simulink model "x5_Click"  (R2024b)
settings: Solver=VariableStepAuto  StartTime=0.0  StopTime=inf  RelTol=1e-3  EnableMultiTasking=on
libraries: simulink x6
(part 1 of 3)
settings Model: Creator=jorgemartins  LastModifiedBy=pinto
settings SolverCC: AlgebraicLoopSolver=TrustRegion
settings DataIOCC: LimitDataPoints=on  ReturnWorkspaceOutputs=off
settings OptimizationCC: LifeSpan=inf
settings DebuggingCC: UnconnectedInputMsg=warning  UnconnectedOutputMsg=warning  UnconnectedLineMsg=warning  AllowSymbolicDim=off  SFUnexpectedBacktrackingDiag=warning  SFNoUnconditionalDefaultTransitionDiag=warning  SFExecutionAtInitializationDiag=none  ArithmeticOperatorsInVariantConditions=warning
settings ModelReferenceCC: EnableRefExpFcnMdlSchedulingChecks=on  PropagateSignalLabelsOutOfModel=off
settings SFSimCC: SimUseLocalCustomCode=off  CustomCodeUndefinedFunction=UseInterfaceOnly
settings RTWCC: RTWUseLocalCustomCode=off  GPUComputeCapability=3.5
settings CodeAppCC: StateflowObjectComments=on
settings GRTTargetCC: TargetLangStandard=C89/C90 (ANSI)
settings ConfigComp: CovMetricSettings=dw  CovSaveCumulativeToWorkspaceVar=on  CovSaveSingleToWorkspaceVar=on  CovExternalEMLEnable=off

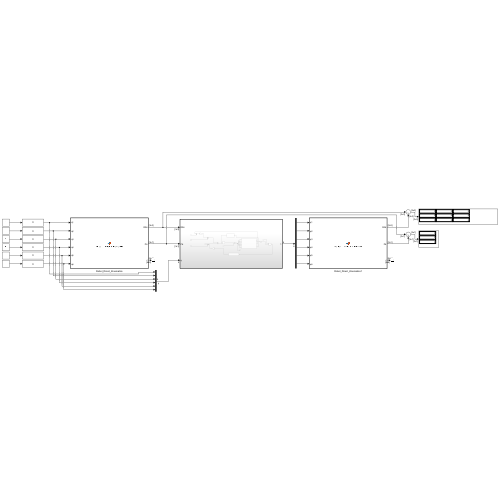
[thumbnail: Simulink's stored preview of the top-level diagram]
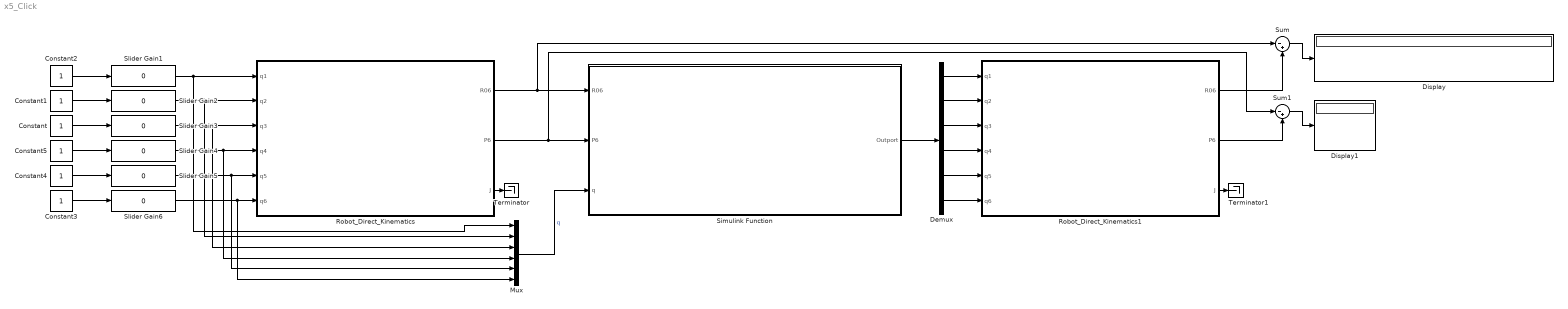
== system x5_Click ==
  Constant{,1..5} (6 alike) : Constant
  Demux : Demux  Outputs=6
  Display : Display
  Display1 : Display
  Mux : Mux  Inputs=6
  Robot_Direct_Kinematics : MATLAB Function  TreatAsAtomicUnit=on
  Robot_Direct_Kinematics1 : MATLAB Function  TreatAsAtomicUnit=on
  Simulink Function : Subsystem  TreatAsAtomicUnit=on
  Slider Gain1 : simulink/Math Operations/Slider Gain  gain=0  low=-3.14  high=0
  Slider Gain{2..4,6} (4 alike) : simulink/Math Operations/Slider Gain  gain=0  low=-3.14  high=3.14
  Slider Gain5 : simulink/Math Operations/Slider Gain  gain=0  low=-3.14  high=0
  Sum : Sum  Inputs=|-+
  Sum1 : Sum  Inputs=|-+
  Terminator : Terminator
  Terminator1 : Terminator
  wires:
  Slider Gain2/1 -> Mux/2, Robot_Direct_Kinematics/2(q2)
  Slider Gain3/1 -> Robot_Direct_Kinematics/3(q3), Mux/3
  Mux/1 -> Simulink Function/3(q)  "q"
  Slider Gain4/1 -> Mux/4, Robot_Direct_Kinematics/4(q4)
  Slider Gain1/1 -> Robot_Direct_Kinematics/1(q1), Mux/1
  Slider Gain5/1 -> Mux/5, Robot_Direct_Kinematics/5(q5)
  Slider Gain6/1 -> Mux/6, Robot_Direct_Kinematics/6(q6)
  Robot_Direct_Kinematics/1(R06) -> Sum/1, Simulink Function/1(R06)
  Robot_Direct_Kinematics/2(P6) -> Sum1/1, Simulink Function/2(P6)
  Constant/1 -> Slider Gain3/1
  Constant1/1 -> Slider Gain2/1
  Constant4/1 -> Slider Gain5/1
  Constant5/1 -> Slider Gain4/1
  Constant3/1 -> Slider Gain6/1
  Constant2/1 -> Slider Gain1/1
  Simulink Function/1(Outport) -> Demux/1
  Demux/1 -> Robot_Direct_Kinematics1/1(q1)
  Demux/2 -> Robot_Direct_Kinematics1/2(q2)
  Demux/3 -> Robot_Direct_Kinematics1/3(q3)
  Demux/4 -> Robot_Direct_Kinematics1/4(q4)
  Demux/5 -> Robot_Direct_Kinematics1/5(q5)
  Demux/6 -> Robot_Direct_Kinematics1/6(q6)
  Robot_Direct_Kinematics1/1(R06) -> Sum/2
  Robot_Direct_Kinematics1/2(P6) -> Sum1/2
  Sum/1 -> Display/1
  Sum1/1 -> Display1/1
  Robot_Direct_Kinematics/3(J) -> Terminator/1
  Robot_Direct_Kinematics1/3(J) -> Terminator1/1

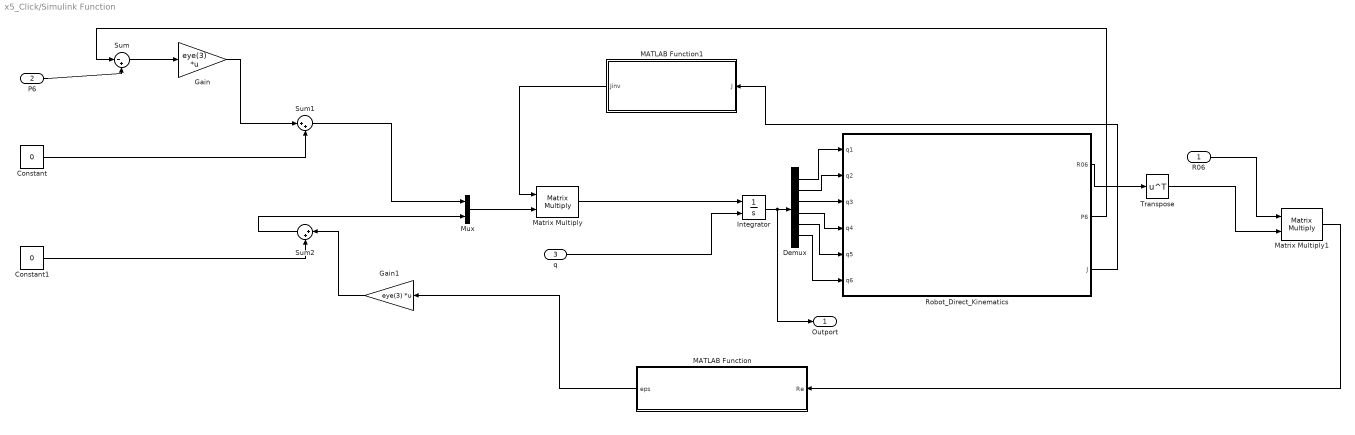
== system x5_Click/Simulink Function ==
  R06 : Inport
  P6 : Inport  Port=2
  q : Inport  Port=3
  Constant : Constant  Value=0
  Constant1 : Constant  Value=0
  Demux : Demux  Outputs=6
  Gain : Gain  Gain=eye(3)  Multiplication=Matrix(K*u) (u vector)
  Gain1 : Gain  Gain=eye(3)  Multiplication=Matrix(K*u) (u vector)
  Integrator : Integrator  InitialConditionSource=external
  MATLAB Function : MATLAB Function  TreatAsAtomicUnit=on
  MATLAB Function1 : MATLAB Function  TreatAsAtomicUnit=on
  Matrix Multiply : Product  Multiplication=Matrix(*)
  Matrix Multiply1 : Product  Multiplication=Matrix(*)
  Mux : Mux  Inputs=2
  Robot_Direct_Kinematics : MATLAB Function  TreatAsAtomicUnit=on
  Sum : Sum  Inputs=|-+
  Sum1 : Sum  Inputs=|++
  Sum2 : Sum  Inputs=|++
  Transpose : Math  Operator=transpose
  Outport : Outport
  wires:
  P6/1 -> Sum/2
  Sum/1 -> Gain/1
  Constant/1 -> Sum1/2
  Gain/1 -> Sum1/1
  Constant1/1 -> Sum2/2
  Gain1/1 -> Sum2/1
  Sum2/1 -> Mux/2
  Sum1/1 -> Mux/1
  Mux/1 -> Matrix Multiply/2
  q/1 -> Integrator/2
  Matrix Multiply/1 -> Integrator/1
  Integrator/1 -> Outport/1, Demux/1
  Demux/1 -> Robot_Direct_Kinematics/1(q1)
  Demux/2 -> Robot_Direct_Kinematics/2(q2)
  Demux/3 -> Robot_Direct_Kinematics/3(q3)
  Demux/4 -> Robot_Direct_Kinematics/4(q4)
  Demux/5 -> Robot_Direct_Kinematics/5(q5)
  Demux/6 -> Robot_Direct_Kinematics/6(q6)
  Robot_Direct_Kinematics/3(J) -> MATLAB Function1/1(J)
  Robot_Direct_Kinematics/2(P6) -> Sum/1
  R06/1 -> Matrix Multiply1/1
  Robot_Direct_Kinematics/1(R06) -> Transpose/1
  Transpose/1 -> Matrix Multiply1/2
  Matrix Multiply1/1 -> MATLAB Function/1(Re)
  MATLAB Function/1(eps) -> Gain1/1
  MATLAB Function1/1(Jinv) -> Matrix Multiply/1

== matlab function x5_Click/Simulink Function/Robot_Direct_Kinematics ==
  data: q1 input; R06 output; q2 input; q3 input; q4 input; q5 input; q6 input; P6 output; J output
function [R06,P6,J] = Robot_Direct_Kinematics(q1,q2,q3,q4,q5,q6)
%#codegen

%    This function was generated by the Symbolic Math Toolbox version 24.2.
%    21-May-2025 19:19:44

% q1 = complex(q1);  % if required to enforce complex operations
% q2 = complex(q2);  % if required to enforce complex operations
% q3 = complex(q3);  % if required to enforce complex operations
% q4 = complex(q4);  % if required to enforce complex operations
% q5 = complex(q5);  % if required to enforce complex operations
% q6 = complex(q6);  % if required to enforce complex operations
et1 = cos(q5).*sin(q1).*sin(q3).*sqrt(sqrt(2.0)+2.0).*(-1.0./2.0)-(cos(q1).*cos(q2).*sin(q4).*sin(q6).*sqrt(-sqrt(2.0)+2.0))./2.0-(cos(q3).*cos(q4).*sin(q1).*sin(q6).*sqrt(-sqrt(2.0)+2.0))./2.0-(cos(q6).*sin(q1).*sin(q3).*sin(q5).*sqrt(-sqrt(2.0)+2.0))./2.0-(cos(q1).*cos(q3).*cos(q5).*sin(q2).*sqrt(sqrt(2.0)+2.0))./2.0-(cos(q1).*cos(q2).*cos(q4).*sin(q5).*sqrt(sqrt(2.0)+2.0))./2.0+(cos(q3).*sin(q1).*sin(q4).*sin(q5).*sqrt(sqrt(2.0)+2.0))./2.0;
et2 = (cos(q1).*cos(q2).*cos(q4).*cos(q5).*cos(q6).*sqrt(-sqrt(2.0)+2.0))./2.0-(cos(q1).*cos(q3).*cos(q6).*sin(q2).*sin(q5).*sqrt(-sqrt(2.0)+2.0))./2.0-(cos(q3).*cos(q5).*cos(q6).*sin(q1).*sin(q4).*sqrt(-sqrt(2.0)+2.0))./2.0+(cos(q1).*cos(q4).*sin(q2).*sin(q3).*sin(q6).*sqrt(-sqrt(2.0)+2.0))./2.0-(cos(q1).*sin(q2).*sin(q3).*sin(q4).*sin(q5).*sqrt(sqrt(2.0)+2.0))./2.0+(cos(q1).*cos(q5).*cos(q6).*sin(q2).*sin(q3).*sin(q4).*sqrt(-sqrt(2.0)+2.0))./2.0;
et3 = cos(q1).*cos(q5).*sin(q3).*sqrt(sqrt(2.0)+2.0).*(-1.0./2.0)-(cos(q1).*cos(q3).*cos(q4).*sin(q6).*sqrt(-sqrt(2.0)+2.0))./2.0-(cos(q1).*cos(q6).*sin(q3).*sin(q5).*sqrt(-sqrt(2.0)+2.0))./2.0+(cos(q2).*sin(q1).*sin(q4).*sin(q6).*sqrt(-sqrt(2.0)+2.0))./2.0+(cos(q3).*cos(q5).*sin(q1).*sin(q2).*sqrt(sqrt(2.0)+2.0))./2.0+(cos(q2).*cos(q4).*sin(q1).*sin(q5).*sqrt(sqrt(2.0)+2.0))./2.0+(cos(q1).*cos(q3).*sin(q4).*sin(q5).*sqrt(sqrt(2.0)+2.0))./2.0-(cos(q2).*cos(q4).*cos(q5).*cos(q6).*sin(q1).*sqrt(-sqrt(2.0)+2.0))./2.0;
et4 = cos(q1).*cos(q3).*cos(q5).*cos(q6).*sin(q4).*sqrt(-sqrt(2.0)+2.0).*(-1.0./2.0)+(cos(q3).*cos(q6).*sin(q1).*sin(q2).*sin(q5).*sqrt(-sqrt(2.0)+2.0))./2.0-(cos(q4).*sin(q1).*sin(q2).*sin(q3).*sin(q6).*sqrt(-sqrt(2.0)+2.0))./2.0+(sin(q1).*sin(q2).*sin(q3).*sin(q4).*sin(q5).*sqrt(sqrt(2.0)+2.0))./2.0-(cos(q5).*cos(q6).*sin(q1).*sin(q2).*sin(q3).*sin(q4).*sqrt(-sqrt(2.0)+2.0))./2.0;
et5 = cos(q5).*sin(q1).*sin(q3).*sqrt(-sqrt(2.0)+2.0).*(-1.0./2.0)-(cos(q1).*cos(q3).*cos(q5).*sin(q2).*sqrt(-sqrt(2.0)+2.0))./2.0-(cos(q1).*cos(q2).*cos(q4).*sin(q5).*sqrt(-sqrt(2.0)+2.0))./2.0+(cos(q3).*sin(q1).*sin(q4).*sin(q5).*sqrt(-sqrt(2.0)+2.0))./2.0+(cos(q1).*cos(q2).*sin(q4).*sin(q6).*sqrt(sqrt(2.0)+2.0))./2.0+(cos(q3).*cos(q4).*sin(q1).*sin(q6).*sqrt(sqrt(2.0)+2.0))./2.0+(cos(q6).*sin(q1).*sin(q3).*sin(q5).*sqrt(sqrt(2.0)+2.0))./2.0;
et6 = cos(q1).*sin(q2).*sin(q3).*sin(q4).*sin(q5).*sqrt(-sqrt(2.0)+2.0).*(-1.0./2.0)-(cos(q1).*cos(q2).*cos(q4).*cos(q5).*cos(q6).*sqrt(sqrt(2.0)+2.0))./2.0+(cos(q1).*cos(q3).*cos(q6).*sin(q2).*sin(q5).*sqrt(sqrt(2.0)+2.0))./2.0+(cos(q3).*cos(q5).*cos(q6).*sin(q1).*sin(q4).*sqrt(sqrt(2.0)+2.0))./2.0-(cos(q1).*cos(q4).*sin(q2).*sin(q3).*sin(q6).*sqrt(sqrt(2.0)+2.0))./2.0-(cos(q1).*cos(q5).*cos(q6).*sin(q2).*sin(q3).*sin(q4).*sqrt(sqrt(2.0)+2.0))./2.0;
et7 = cos(q1).*cos(q5).*sin(q3).*sqrt(-sqrt(2.0)+2.0).*(-1.0./2.0)+(cos(q3).*cos(q5).*sin(q1).*sin(q2).*sqrt(-sqrt(2.0)+2.0))./2.0+(cos(q2).*cos(q4).*sin(q1).*sin(q5).*sqrt(-sqrt(2.0)+2.0))./2.0+(cos(q1).*cos(q3).*sin(q4).*sin(q5).*sqrt(-sqrt(2.0)+2.0))./2.0+(cos(q1).*cos(q3).*cos(q4).*sin(q6).*sqrt(sqrt(2.0)+2.0))./2.0+(cos(q1).*cos(q6).*sin(q3).*sin(q5).*sqrt(sqrt(2.0)+2.0))./2.0-(cos(q2).*sin(q1).*sin(q4).*sin(q6).*sqrt(sqrt(2.0)+2.0))./2.0;
et8 = (sin(q1).*sin(q2).*sin(q3).*sin(q4).*sin(q5).*sqrt(-sqrt(2.0)+2.0))./2.0+(cos(q2).*cos(q4).*cos(q5).*cos(q6).*sin(q1).*sqrt(sqrt(2.0)+2.0))./2.0+(cos(q1).*cos(q3).*cos(q5).*cos(q6).*sin(q4).*sqrt(sqrt(2.0)+2.0))./2.0-(cos(q3).*cos(q6).*sin(q1).*sin(q2).*sin(q5).*sqrt(sqrt(2.0)+2.0))./2.0+(cos(q4).*sin(q1).*sin(q2).*sin(q3).*sin(q6).*sqrt(sqrt(2.0)+2.0))./2.0+(cos(q5).*cos(q6).*sin(q1).*sin(q2).*sin(q3).*sin(q4).*sqrt(sqrt(2.0)+2.0))./2.0;
mt1 = [cos(q1).*cos(q3).*cos(q4).*cos(q6)-cos(q2).*cos(q6).*sin(q1).*sin(q4)-cos(q1).*sin(q3).*sin(q5).*sin(q6)-cos(q2).*cos(q4).*cos(q5).*sin(q1).*sin(q6)-cos(q1).*cos(q3).*cos(q5).*sin(q4).*sin(q6)+cos(q4).*cos(q6).*sin(q1).*sin(q2).*sin(q3)+cos(q3).*sin(q1).*sin(q2).*sin(q5).*sin(q6)-cos(q5).*sin(q1).*sin(q2).*sin(q3).*sin(q4).*sin(q6),cos(q1).*cos(q2).*cos(q6).*sin(q4)+cos(q3).*cos(q4).*cos(q6).*sin(q1)-sin(q1).*sin(q3).*sin(q5).*sin(q6)+cos(q1).*cos(q2).*cos(q4).*cos(q5).*sin(q6)-cos(q1).*cos(q4).*cos(q6).*sin(q2).*sin(q3)-cos(q1).*cos(q3).*sin(q2).*sin(q5).*sin(q6)-cos(q3).*cos(q5).*sin(q1).*sin(q4).*sin(q6)+cos(q1).*cos(q5).*sin(q2).*sin(q3).*sin(q4).*sin(q6)];
mt2 = [cos(q6).*sin(q2).*sin(q4)+cos(q2).*cos(q4).*cos(q6).*sin(q3)+cos(q2).*cos(q3).*sin(q5).*sin(q6)+cos(q4).*cos(q5).*sin(q2).*sin(q6)-cos(q2).*cos(q5).*sin(q3).*sin(q4).*sin(q6),et3+et4,et1+et2];
mt3 = [cos(q4).*sin(q2).*sin(q5).*sqrt(sqrt(2.0)+2.0).*(-1.0./2.0)-(sin(q2).*sin(q4).*sin(q6).*sqrt(-sqrt(2.0)+2.0))./2.0+(cos(q2).*cos(q3).*cos(q5).*sqrt(sqrt(2.0)+2.0))./2.0+(cos(q2).*cos(q3).*cos(q6).*sin(q5).*sqrt(-sqrt(2.0)+2.0))./2.0+(cos(q4).*cos(q5).*cos(q6).*sin(q2).*sqrt(-sqrt(2.0)+2.0))./2.0-(cos(q2).*cos(q4).*sin(q3).*sin(q6).*sqrt(-sqrt(2.0)+2.0))./2.0+(cos(q2).*sin(q3).*sin(q4).*sin(q5).*sqrt(sqrt(2.0)+2.0))./2.0-(cos(q2).*cos(q5).*cos(q6).*sin(q3).*sin(q4).*sqrt(-sqrt(2.0)+2.0))./2.0];
mt4 = [et7+et8,et5+et6,(sin(q2).*sin(q4).*sin(q6).*sqrt(sqrt(2.0)+2.0))./2.0+(cos(q2).*cos(q3).*cos(q5).*sqrt(-sqrt(2.0)+2.0))./2.0-(cos(q4).*sin(q2).*sin(q5).*sqrt(-sqrt(2.0)+2.0))./2.0+(cos(q2).*sin(q3).*sin(q4).*sin(q5).*sqrt(-sqrt(2.0)+2.0))./2.0-(cos(q2).*cos(q3).*cos(q6).*sin(q5).*sqrt(sqrt(2.0)+2.0))./2.0-(cos(q4).*cos(q5).*cos(q6).*sin(q2).*sqrt(sqrt(2.0)+2.0))./2.0+(cos(q2).*cos(q4).*sin(q3).*sin(q6).*sqrt(sqrt(2.0)+2.0))./2.0+(cos(q2).*cos(q5).*cos(q6).*sin(q3).*sin(q4).*sqrt(sqrt(2.0)+2.0))./2.0];
R06 = reshape([mt1,mt2,mt3,mt4],3,3);
if nargout > 1
    et9 = sin(q2).*(-2.0./5.0)+(cos(q4).*sin(q2))./1.0e+1+(sin(q2).*sin(q4))./2.0+(cos(q2).*cos(q3).*cos(q5))./1.0e+1+(cos(q2).*cos(q4).*sin(q3))./2.0-(cos(q2).*sin(q3).*sin(q4))./1.0e+1-(cos(q4).*sin(q2).*sin(q5))./1.0e+1+sin(q2).*sin(q4).*sin(q6).*sqrt(sqrt(2.0)+2.0).*(3.0./4.0e+1)+cos(q2).*cos(q3).*cos(q5).*sqrt(-sqrt(2.0)+2.0).*(3.0./4.0e+1)-cos(q4).*sin(q2).*sin(q5).*sqrt(-sqrt(2.0)+2.0).*(3.0./4.0e+1)+(cos(q2).*sin(q3).*sin(q4).*sin(q5))./1.0e+1+cos(q2).*sin(q3).*sin(q4).*sin(q5).*sqrt(-sqrt(2.0)+2.0).*(3.0./4.0e+1);
    et10 = cos(q2).*cos(q3).*cos(q6).*sin(q5).*sqrt(sqrt(2.0)+2.0).*(-3.0./4.0e+1)-cos(q4).*cos(q5).*cos(q6).*sin(q2).*sqrt(sqrt(2.0)+2.0).*(3.0./4.0e+1)+cos(q2).*cos(q4).*sin(q3).*sin(q6).*sqrt(sqrt(2.0)+2.0).*(3.0./4.0e+1)+cos(q2).*cos(q5).*cos(q6).*sin(q3).*sin(q4).*sqrt(sqrt(2.0)+2.0).*(3.0./4.0e+1);
    et11 = cos(q1).*cos(q2).*(-2.0./5.0)+(cos(q1).*cos(q2).*cos(q4))./1.0e+1+(cos(q1).*cos(q2).*sin(q4))./2.0+(cos(q3).*cos(q4).*sin(q1))./2.0-(cos(q3).*sin(q1).*sin(q4))./1.0e+1-(cos(q5).*sin(q1).*sin(q3))./1.0e+1-cos(q5).*sin(q1).*sin(q3).*sqrt(-sqrt(2.0)+2.0).*(3.0./4.0e+1)-(cos(q1).*cos(q3).*cos(q5).*sin(q2))./1.0e+1-(cos(q1).*cos(q2).*cos(q4).*sin(q5))./1.0e+1-(cos(q1).*cos(q4).*sin(q2).*sin(q3))./2.0+(cos(q1).*sin(q2).*sin(q3).*sin(q4))./1.0e+1+(cos(q3).*sin(q1).*sin(q4).*sin(q5))./1.0e+1-cos(q1).*cos(q3).*cos(q5).*sin(q2).*sqrt(-sqrt(2.0)+2.0).*(3.0./4.0e+1);
    et12 = cos(q1).*cos(q2).*cos(q4).*sin(q5).*sqrt(-sqrt(2.0)+2.0).*(-3.0./4.0e+1)+cos(q3).*sin(q1).*sin(q4).*sin(q5).*sqrt(-sqrt(2.0)+2.0).*(3.0./4.0e+1)-(cos(q1).*sin(q2).*sin(q3).*sin(q4).*sin(q5))./1.0e+1+cos(q1).*cos(q2).*sin(q4).*sin(q6).*sqrt(sqrt(2.0)+2.0).*(3.0./4.0e+1)+cos(q3).*cos(q4).*sin(q1).*sin(q6).*sqrt(sqrt(2.0)+2.0).*(3.0./4.0e+1)+cos(q6).*sin(q1).*sin(q3).*sin(q5).*sqrt(sqrt(2.0)+2.0).*(3.0./4.0e+1)-cos(q1).*sin(q2).*sin(q3).*sin(q4).*sin(q5).*sqrt(-sqrt(2.0)+2.0).*(3.0./4.0e+1)-cos(q1).*cos(q2).*cos(q4).*cos(q5).*cos(q6).*sqrt(sqrt(2.0)+2.0).*(3.0./4.0e+1);
    et13 = cos(q1).*cos(q3).*cos(q6).*sin(q2).*sin(q5).*sqrt(sqrt(2.0)+2.0).*(3.0./4.0e+1)+cos(q3).*cos(q5).*cos(q6).*sin(q1).*sin(q4).*sqrt(sqrt(2.0)+2.0).*(3.0./4.0e+1)-cos(q1).*cos(q4).*sin(q2).*sin(q3).*sin(q6).*sqrt(sqrt(2.0)+2.0).*(3.0./4.0e+1)-cos(q1).*cos(q5).*cos(q6).*sin(q2).*sin(q3).*sin(q4).*sqrt(sqrt(2.0)+2.0).*(3.0./4.0e+1);
    et14 = cos(q2).*sin(q1).*(2.0./5.0)+(cos(q1).*cos(q3).*cos(q4))./2.0-(cos(q2).*cos(q4).*sin(q1))./1.0e+1-(cos(q1).*cos(q3).*sin(q4))./1.0e+1-(cos(q1).*cos(q5).*sin(q3))./1.0e+1-(cos(q2).*sin(q1).*sin(q4))./2.0-cos(q1).*cos(q5).*sin(q3).*sqrt(-sqrt(2.0)+2.0).*(3.0./4.0e+1)+(cos(q3).*cos(q5).*sin(q1).*sin(q2))./1.0e+1+(cos(q2).*cos(q4).*sin(q1).*sin(q5))./1.0e+1+(cos(q1).*cos(q3).*sin(q4).*sin(q5))./1.0e+1+(cos(q4).*sin(q1).*sin(q2).*sin(q3))./2.0-(sin(q1).*sin(q2).*sin(q3).*sin(q4))./1.0e+1+cos(q3).*cos(q5).*sin(q1).*sin(q2).*sqrt(-sqrt(2.0)+2.0).*(3.0./4.0e+1);
    et15 = cos(q2).*cos(q4).*sin(q1).*sin(q5).*sqrt(-sqrt(2.0)+2.0).*(3.0./4.0e+1)+cos(q1).*cos(q3).*sin(q4).*sin(q5).*sqrt(-sqrt(2.0)+2.0).*(3.0./4.0e+1)+(sin(q1).*sin(q2).*sin(q3).*sin(q4).*sin(q5))./1.0e+1+cos(q1).*cos(q3).*cos(q4).*sin(q6).*sqrt(sqrt(2.0)+2.0).*(3.0./4.0e+1)+cos(q1).*cos(q6).*sin(q3).*sin(q5).*sqrt(sqrt(2.0)+2.0).*(3.0./4.0e+1)-cos(q2).*sin(q1).*sin(q4).*sin(q6).*sqrt(sqrt(2.0)+2.0).*(3.0./4.0e+1)+sin(q1).*sin(q2).*sin(q3).*sin(q4).*sin(q5).*sqrt(-sqrt(2.0)+2.0).*(3.0./4.0e+1)+cos(q2).*cos(q4).*cos(q5).*cos(q6).*sin(q1).*sqrt(sqrt(2.0)+2.0).*(3.0./4.0e+1);
    et16 = cos(q1).*cos(q3).*cos(q5).*cos(q6).*sin(q4).*sqrt(sqrt(2.0)+2.0).*(3.0./4.0e+1)-cos(q3).*cos(q6).*sin(q1).*sin(q2).*sin(q5).*sqrt(sqrt(2.0)+2.0).*(3.0./4.0e+1)+cos(q4).*sin(q1).*sin(q2).*sin(q3).*sin(q6).*sqrt(sqrt(2.0)+2.0).*(3.0./4.0e+1)+cos(q5).*cos(q6).*sin(q1).*sin(q2).*sin(q3).*sin(q4).*sqrt(sqrt(2.0)+2.0).*(3.0./4.0e+1);
    P6 = [et14+et15+et16;et11+et12+et13;et9+et10];
end
if nargout > 2
    et17 = cos(q2).*sin(q1).*(2.0./5.0)+(cos(q1).*cos(q3).*cos(q4))./2.0-(cos(q2).*cos(q4).*sin(q1))./1.0e+1-(cos(q1).*cos(q3).*sin(q4))./1.0e+1-(cos(q1).*cos(q5).*sin(q3))./1.0e+1-(cos(q2).*sin(q1).*sin(q4))./2.0-cos(q1).*cos(q5).*sin(q3).*sqrt(-sqrt(2.0)+2.0).*(3.0./4.0e+1)+(cos(q3).*cos(q5).*sin(q1).*sin(q2))./1.0e+1+(cos(q2).*cos(q4).*sin(q1).*sin(q5))./1.0e+1+(cos(q1).*cos(q3).*sin(q4).*sin(q5))./1.0e+1+(cos(q4).*sin(q1).*sin(q2).*sin(q3))./2.0-(sin(q1).*sin(q2).*sin(q3).*sin(q4))./1.0e+1+cos(q3).*cos(q5).*sin(q1).*sin(q2).*sqrt(-sqrt(2.0)+2.0).*(3.0./4.0e+1);
    et18 = cos(q2).*cos(q4).*sin(q1).*sin(q5).*sqrt(-sqrt(2.0)+2.0).*(3.0./4.0e+1)+cos(q1).*cos(q3).*sin(q4).*sin(q5).*sqrt(-sqrt(2.0)+2.0).*(3.0./4.0e+1)+(sin(q1).*sin(q2).*sin(q3).*sin(q4).*sin(q5))./1.0e+1+cos(q1).*cos(q3).*cos(q4).*sin(q6).*sqrt(sqrt(2.0)+2.0).*(3.0./4.0e+1)+cos(q1).*cos(q6).*sin(q3).*sin(q5).*sqrt(sqrt(2.0)+2.0).*(3.0./4.0e+1)-cos(q2).*sin(q1).*sin(q4).*sin(q6).*sqrt(sqrt(2.0)+2.0).*(3.0./4.0e+1)+sin(q1).*sin(q2).*sin(q3).*sin(q4).*sin(q5).*sqrt(-sqrt(2.0)+2.0).*(3.0./4.0e+1)+cos(q2).*cos(q4).*cos(q5).*cos(q6).*sin(q1).*sqrt(sqrt(2.0)+2.0).*(3.0./4.0e+1);
    et19 = cos(q1).*cos(q3).*cos(q5).*cos(q6).*sin(q4).*sqrt(sqrt(2.0)+2.0).*(3.0./4.0e+1)-cos(q3).*cos(q6).*sin(q1).*sin(q2).*sin(q5).*sqrt(sqrt(2.0)+2.0).*(3.0./4.0e+1)+cos(q4).*sin(q1).*sin(q2).*sin(q3).*sin(q6).*sqrt(sqrt(2.0)+2.0).*(3.0./4.0e+1)+cos(q5).*cos(q6).*sin(q1).*sin(q2).*sin(q3).*sin(q4).*sqrt(sqrt(2.0)+2.0).*(3.0./4.0e+1);
    et20 = cos(q1).*cos(q2).*(2.0./5.0)-(cos(q1).*cos(q2).*cos(q4))./1.0e+1-(cos(q1).*cos(q2).*sin(q4))./2.0-(cos(q3).*cos(q4).*sin(q1))./2.0+(cos(q3).*sin(q1).*sin(q4))./1.0e+1+(cos(q5).*sin(q1).*sin(q3))./1.0e+1+cos(q5).*sin(q1).*sin(q3).*sqrt(-sqrt(2.0)+2.0).*(3.0./4.0e+1)+(cos(q1).*cos(q3).*cos(q5).*sin(q2))./1.0e+1+(cos(q1).*cos(q2).*cos(q4).*sin(q5))./1.0e+1+(cos(q1).*cos(q4).*sin(q2).*sin(q3))./2.0-(cos(q1).*sin(q2).*sin(q3).*sin(q4))./1.0e+1-(cos(q3).*sin(q1).*sin(q4).*sin(q5))./1.0e+1+cos(q1).*cos(q3).*cos(q5).*sin(q2).*sqrt(-sqrt(2.0)+2.0).*(3.0./4.0e+1);
    et21 = cos(q1).*cos(q2).*cos(q4).*sin(q5).*sqrt(-sqrt(2.0)+2.0).*(3.0./4.0e+1)-cos(q3).*sin(q1).*sin(q4).*sin(q5).*sqrt(-sqrt(2.0)+2.0).*(3.0./4.0e+1)+(cos(q1).*sin(q2).*sin(q3).*sin(q4).*sin(q5))./1.0e+1-cos(q1).*cos(q2).*sin(q4).*sin(q6).*sqrt(sqrt(2.0)+2.0).*(3.0./4.0e+1)-cos(q3).*cos(q4).*sin(q1).*sin(q6).*sqrt(sqrt(2.0)+2.0).*(3.0./4.0e+1)-cos(q6).*sin(q1).*sin(q3).*sin(q5).*sqrt(sqrt(2.0)+2.0).*(3.0./4.0e+1)+cos(q1).*sin(q2).*sin(q3).*sin(q4).*sin(q5).*sqrt(-sqrt(2.0)+2.0).*(3.0./4.0e+1)+cos(q1).*cos(q2).*cos(q4).*cos(q5).*cos(q6).*sqrt(sqrt(2.0)+2.0).*(3.0./4.0e+1);
    et22 = cos(q1).*cos(q3).*cos(q6).*sin(q2).*sin(q5).*sqrt(sqrt(2.0)+2.0).*(-3.0./4.0e+1)-cos(q3).*cos(q5).*cos(q6).*sin(q1).*sin(q4).*sqrt(sqrt(2.0)+2.0).*(3.0./4.0e+1)+cos(q1).*cos(q4).*sin(q2).*sin(q3).*sin(q6).*sqrt(sqrt(2.0)+2.0).*(3.0./4.0e+1)+cos(q1).*cos(q5).*cos(q6).*sin(q2).*sin(q3).*sin(q4).*sqrt(sqrt(2.0)+2.0).*(3.0./4.0e+1);
    et23 = cos(q2).*(-2.0./5.0)+(cos(q2).*cos(q4))./1.0e+1+(cos(q2).*sin(q4))./2.0+(sin(q2).*sin(q3).*sin(q4))./1.0e+1-(cos(q3).*cos(q5).*sin(q2))./1.0e+1-(cos(q2).*cos(q4).*sin(q5))./1.0e+1-(cos(q4).*sin(q2).*sin(q3))./2.0+cos(q2).*sin(q4).*sin(q6).*sqrt(sqrt(2.0)+2.0).*(3.0./4.0e+1)-cos(q3).*cos(q5).*sin(q2).*sqrt(-sqrt(2.0)+2.0).*(3.0./4.0e+1)-cos(q2).*cos(q4).*sin(q5).*sqrt(-sqrt(2.0)+2.0).*(3.0./4.0e+1)-(sin(q2).*sin(q3).*sin(q4).*sin(q5))./1.0e+1-sin(q2).*sin(q3).*sin(q4).*sin(q5).*sqrt(-sqrt(2.0)+2.0).*(3.0./4.0e+1);
    et24 = cos(q2).*cos(q4).*cos(q5).*cos(q6).*sqrt(sqrt(2.0)+2.0).*(-3.0./4.0e+1)+cos(q3).*cos(q6).*sin(q2).*sin(q5).*sqrt(sqrt(2.0)+2.0).*(3.0./4.0e+1)-cos(q4).*sin(q2).*sin(q3).*sin(q6).*sqrt(sqrt(2.0)+2.0).*(3.0./4.0e+1)-cos(q5).*cos(q6).*sin(q2).*sin(q3).*sin(q4).*sqrt(sqrt(2.0)+2.0).*(3.0./4.0e+1);
    et25 = sin(q2).*-1.6e+1+cos(q4).*sin(q2).*4.0+sin(q2).*sin(q4).*2.0e+1+cos(q2).*cos(q3).*cos(q5).*4.0+cos(q2).*cos(q4).*sin(q3).*2.0e+1-cos(q2).*sin(q3).*sin(q4).*4.0-cos(q4).*sin(q2).*sin(q5).*4.0+sin(q2).*sin(q4).*sin(q6).*sqrt(sqrt(2.0)+2.0).*3.0+cos(q2).*cos(q3).*cos(q5).*sqrt(-sqrt(2.0)+2.0).*3.0-cos(q4).*sin(q2).*sin(q5).*sqrt(-sqrt(2.0)+2.0).*3.0+cos(q2).*sin(q3).*sin(q4).*sin(q5).*4.0+cos(q2).*sin(q3).*sin(q4).*sin(q5).*sqrt(-sqrt(2.0)+2.0).*3.0-cos(q2).*cos(q3).*cos(q6).*sin(q5).*sqrt(sqrt(2.0)+2.0).*3.0-cos(q4).*cos(q5).*cos(q6).*sin(q2).*sqrt(sqrt(2.0)+2.0).*3.0;
    et26 = cos(q2).*cos(q4).*sin(q3).*sin(q6).*sqrt(sqrt(2.0)+2.0).*3.0+cos(q2).*cos(q5).*cos(q6).*sin(q3).*sin(q4).*sqrt(sqrt(2.0)+2.0).*3.0;
    et27 = sin(q2).*-1.6e+1+cos(q4).*sin(q2).*4.0+sin(q2).*sin(q4).*2.0e+1+cos(q2).*cos(q3).*cos(q5).*4.0+cos(q2).*cos(q4).*sin(q3).*2.0e+1-cos(q2).*sin(q3).*sin(q4).*4.0-cos(q4).*sin(q2).*sin(q5).*4.0+sin(q2).*sin(q4).*sin(q6).*sqrt(sqrt(2.0)+2.0).*3.0+cos(q2).*cos(q3).*cos(q5).*sqrt(-sqrt(2.0)+2.0).*3.0-cos(q4).*sin(q2).*sin(q5).*sqrt(-sqrt(2.0)+2.0).*3.0+cos(q2).*sin(q3).*sin(q4).*sin(q5).*4.0+cos(q2).*sin(q3).*sin(q4).*sin(q5).*sqrt(-sqrt(2.0)+2.0).*3.0-cos(q2).*cos(q3).*cos(q6).*sin(q5).*sqrt(sqrt(2.0)+2.0).*3.0-cos(q4).*cos(q5).*cos(q6).*sin(q2).*sqrt(sqrt(2.0)+2.0).*3.0;
    et28 = cos(q2).*cos(q4).*sin(q3).*sin(q6).*sqrt(sqrt(2.0)+2.0).*3.0+cos(q2).*cos(q5).*cos(q6).*sin(q3).*sin(q4).*sqrt(sqrt(2.0)+2.0).*3.0;
    et29 = (sin(q1).*sin(q3).*sin(q4))./1.0e+1-(cos(q3).*cos(q5).*sin(q1))./1.0e+1-(cos(q4).*sin(q1).*sin(q3))./2.0-cos(q3).*cos(q5).*sin(q1).*sqrt(-sqrt(2.0)+2.0).*(3.0./4.0e+1)-(cos(q1).*cos(q3).*cos(q4).*sin(q2))./2.0+(cos(q1).*cos(q3).*sin(q2).*sin(q4))./1.0e+1+(cos(q1).*cos(q5).*sin(q2).*sin(q3))./1.0e+1-(sin(q1).*sin(q3).*sin(q4).*sin(q5))./1.0e+1+cos(q1).*cos(q5).*sin(q2).*sin(q3).*sqrt(-sqrt(2.0)+2.0).*(3.0./4.0e+1)-sin(q1).*sin(q3).*sin(q4).*sin(q5).*sqrt(-sqrt(2.0)+2.0).*(3.0./4.0e+1)-(cos(q1).*cos(q3).*sin(q2).*sin(q4).*sin(q5))./1.0e+1;
    et30 = cos(q3).*cos(q6).*sin(q1).*sin(q5).*sqrt(sqrt(2.0)+2.0).*(3.0./4.0e+1)-cos(q4).*sin(q1).*sin(q3).*sin(q6).*sqrt(sqrt(2.0)+2.0).*(3.0./4.0e+1)-cos(q1).*cos(q3).*sin(q2).*sin(q4).*sin(q5).*sqrt(-sqrt(2.0)+2.0).*(3.0./4.0e+1)-cos(q1).*cos(q3).*cos(q4).*sin(q2).*sin(q6).*sqrt(sqrt(2.0)+2.0).*(3.0./4.0e+1)-cos(q1).*cos(q6).*sin(q2).*sin(q3).*sin(q5).*sqrt(sqrt(2.0)+2.0).*(3.0./4.0e+1)-cos(q5).*cos(q6).*sin(q1).*sin(q3).*sin(q4).*sqrt(sqrt(2.0)+2.0).*(3.0./4.0e+1)-cos(q1).*cos(q3).*cos(q5).*cos(q6).*sin(q2).*sin(q4).*sqrt(sqrt(2.0)+2.0).*(3.0./4.0e+1);
    et31 = cos(q1).*cos(q3).*cos(q5).*(-1.0./1.0e+1)-(cos(q1).*cos(q4).*sin(q3))./2.0+(cos(q1).*sin(q3).*sin(q4))./1.0e+1-cos(q1).*cos(q3).*cos(q5).*sqrt(-sqrt(2.0)+2.0).*(3.0./4.0e+1)+(cos(q3).*cos(q4).*sin(q1).*sin(q2))./2.0-(cos(q3).*sin(q1).*sin(q2).*sin(q4))./1.0e+1-(cos(q5).*sin(q1).*sin(q2).*sin(q3))./1.0e+1-(cos(q1).*sin(q3).*sin(q4).*sin(q5))./1.0e+1-cos(q5).*sin(q1).*sin(q2).*sin(q3).*sqrt(-sqrt(2.0)+2.0).*(3.0./4.0e+1)-cos(q1).*sin(q3).*sin(q4).*sin(q5).*sqrt(-sqrt(2.0)+2.0).*(3.0./4.0e+1)+(cos(q3).*sin(q1).*sin(q2).*sin(q4).*sin(q5))./1.0e+1;
    et32 = cos(q1).*cos(q3).*cos(q6).*sin(q5).*sqrt(sqrt(2.0)+2.0).*(3.0./4.0e+1)-cos(q1).*cos(q4).*sin(q3).*sin(q6).*sqrt(sqrt(2.0)+2.0).*(3.0./4.0e+1)+cos(q3).*sin(q1).*sin(q2).*sin(q4).*sin(q5).*sqrt(-sqrt(2.0)+2.0).*(3.0./4.0e+1)-cos(q1).*cos(q5).*cos(q6).*sin(q3).*sin(q4).*sqrt(sqrt(2.0)+2.0).*(3.0./4.0e+1)+cos(q3).*cos(q4).*sin(q1).*sin(q2).*sin(q6).*sqrt(sqrt(2.0)+2.0).*(3.0./4.0e+1)+cos(q6).*sin(q1).*sin(q2).*sin(q3).*sin(q5).*sqrt(sqrt(2.0)+2.0).*(3.0./4.0e+1)+cos(q3).*cos(q5).*cos(q6).*sin(q1).*sin(q2).*sin(q4).*sqrt(sqrt(2.0)+2.0).*(3.0./4.0e+1);
    et33 = (cos(q4).*sin(q2))./2.0-(sin(q2).*sin(q4))./1.0e+1+(sin(q2).*sin(q4).*sin(q5))./1.0e+1-(cos(q2).*cos(q4).*sin(q3))./1.0e+1-(cos(q2).*sin(q3).*sin(q4))./2.0+cos(q4).*sin(q2).*sin(q6).*sqrt(sqrt(2.0)+2.0).*(3.0./4.0e+1)+sin(q2).*sin(q4).*sin(q5).*sqrt(-sqrt(2.0)+2.0).*(3.0./4.0e+1)+(cos(q2).*cos(q4).*sin(q3).*sin(q5))./1.0e+1+cos(q2).*cos(q4).*sin(q3).*sin(q5).*sqrt(-sqrt(2.0)+2.0).*(3.0./4.0e+1)+cos(q5).*cos(q6).*sin(q2).*sin(q4).*sqrt(sqrt(2.0)+2.0).*(3.0./4.0e+1)-cos(q2).*sin(q3).*sin(q4).*sin(q6).*sqrt(sqrt(2.0)+2.0).*(3.0./4.0e+1);
    et34 = cos(q2).*cos(q4).*cos(q5).*cos(q6).*sin(q3).*sqrt(sqrt(2.0)+2.0).*(3.0./4.0e+1);
    et35 = (cos(q1).*cos(q2).*cos(q4))./2.0-(cos(q1).*cos(q2).*sin(q4))./1.0e+1-(cos(q3).*cos(q4).*sin(q1))./1.0e+1-(cos(q3).*sin(q1).*sin(q4))./2.0+(cos(q1).*cos(q4).*sin(q2).*sin(q3))./1.0e+1+(cos(q1).*cos(q2).*sin(q4).*sin(q5))./1.0e+1+(cos(q3).*cos(q4).*sin(q1).*sin(q5))./1.0e+1+(cos(q1).*sin(q2).*sin(q3).*sin(q4))./2.0+cos(q1).*cos(q2).*sin(q4).*sin(q5).*sqrt(-sqrt(2.0)+2.0).*(3.0./4.0e+1)+cos(q3).*cos(q4).*sin(q1).*sin(q5).*sqrt(-sqrt(2.0)+2.0).*(3.0./4.0e+1)-(cos(q1).*cos(q4).*sin(q2).*sin(q3).*sin(q5))./1.0e+1+cos(q1).*cos(q2).*cos(q4).*sin(q6).*sqrt(sqrt(2.0)+2.0).*(3.0./4.0e+1);
    et36 = cos(q3).*sin(q1).*sin(q4).*sin(q6).*sqrt(sqrt(2.0)+2.0).*(-3.0./4.0e+1)-cos(q1).*cos(q4).*sin(q2).*sin(q3).*sin(q5).*sqrt(-sqrt(2.0)+2.0).*(3.0./4.0e+1)+cos(q1).*cos(q2).*cos(q5).*cos(q6).*sin(q4).*sqrt(sqrt(2.0)+2.0).*(3.0./4.0e+1)+cos(q3).*cos(q4).*cos(q5).*cos(q6).*sin(q1).*sqrt(sqrt(2.0)+2.0).*(3.0./4.0e+1)+cos(q1).*sin(q2).*sin(q3).*sin(q4).*sin(q6).*sqrt(sqrt(2.0)+2.0).*(3.0./4.0e+1)-cos(q1).*cos(q4).*cos(q5).*cos(q6).*sin(q2).*sin(q3).*sqrt(sqrt(2.0)+2.0).*(3.0./4.0e+1);
    et37 = cos(q1).*cos(q3).*cos(q4).*(-1.0./1.0e+1)-(cos(q2).*cos(q4).*sin(q1))./2.0-(cos(q1).*cos(q3).*sin(q4))./2.0+(cos(q2).*sin(q1).*sin(q4))./1.0e+1+(cos(q1).*cos(q3).*cos(q4).*sin(q5))./1.0e+1-(cos(q4).*sin(q1).*sin(q2).*sin(q3))./1.0e+1-(cos(q2).*sin(q1).*sin(q4).*sin(q5))./1.0e+1-(sin(q1).*sin(q2).*sin(q3).*sin(q4))./2.0+cos(q1).*cos(q3).*cos(q4).*sin(q5).*sqrt(-sqrt(2.0)+2.0).*(3.0./4.0e+1)-cos(q2).*sin(q1).*sin(q4).*sin(q5).*sqrt(-sqrt(2.0)+2.0).*(3.0./4.0e+1)+(cos(q4).*sin(q1).*sin(q2).*sin(q3).*sin(q5))./1.0e+1-cos(q2).*cos(q4).*sin(q1).*sin(q6).*sqrt(sqrt(2.0)+2.0).*(3.0./4.0e+1);
    et38 = cos(q1).*cos(q3).*sin(q4).*sin(q6).*sqrt(sqrt(2.0)+2.0).*(-3.0./4.0e+1)+cos(q4).*sin(q1).*sin(q2).*sin(q3).*sin(q5).*sqrt(-sqrt(2.0)+2.0).*(3.0./4.0e+1)+cos(q1).*cos(q3).*cos(q4).*cos(q5).*cos(q6).*sqrt(sqrt(2.0)+2.0).*(3.0./4.0e+1)-cos(q2).*cos(q5).*cos(q6).*sin(q1).*sin(q4).*sqrt(sqrt(2.0)+2.0).*(3.0./4.0e+1)-sin(q1).*sin(q2).*sin(q3).*sin(q4).*sin(q6).*sqrt(sqrt(2.0)+2.0).*(3.0./4.0e+1)+cos(q4).*cos(q5).*cos(q6).*sin(q1).*sin(q2).*sin(q3).*sqrt(sqrt(2.0)+2.0).*(3.0./4.0e+1);
    et39 = (sin(q1).*sin(q3).*sin(q5))./1.0e+1+sin(q1).*sin(q3).*sin(q5).*sqrt(-sqrt(2.0)+2.0).*(3.0./4.0e+1)-(cos(q1).*cos(q2).*cos(q4).*cos(q5))./1.0e+1+(cos(q1).*cos(q3).*sin(q2).*sin(q5))./1.0e+1+(cos(q3).*cos(q5).*sin(q1).*sin(q4))./1.0e+1-cos(q1).*cos(q2).*cos(q4).*cos(q5).*sqrt(-sqrt(2.0)+2.0).*(3.0./4.0e+1)+cos(q1).*cos(q3).*sin(q2).*sin(q5).*sqrt(-sqrt(2.0)+2.0).*(3.0./4.0e+1)+cos(q3).*cos(q5).*sin(q1).*sin(q4).*sqrt(-sqrt(2.0)+2.0).*(3.0./4.0e+1)-(cos(q1).*cos(q5).*sin(q2).*sin(q3).*sin(q4))./1.0e+1+cos(q5).*cos(q6).*sin(q1).*sin(q3).*sqrt(sqrt(2.0)+2.0).*(3.0./4.0e+1);
    et40 = cos(q1).*cos(q5).*sin(q2).*sin(q3).*sin(q4).*sqrt(-sqrt(2.0)+2.0).*(-3.0./4.0e+1)+cos(q1).*cos(q3).*cos(q5).*cos(q6).*sin(q2).*sqrt(sqrt(2.0)+2.0).*(3.0./4.0e+1)+cos(q1).*cos(q2).*cos(q4).*cos(q6).*sin(q5).*sqrt(sqrt(2.0)+2.0).*(3.0./4.0e+1)-cos(q3).*cos(q6).*sin(q1).*sin(q4).*sin(q5).*sqrt(sqrt(2.0)+2.0).*(3.0./4.0e+1)+cos(q1).*cos(q6).*sin(q2).*sin(q3).*sin(q4).*sin(q5).*sqrt(sqrt(2.0)+2.0).*(3.0./4.0e+1);
    et41 = (cos(q1).*sin(q3).*sin(q5))./1.0e+1+cos(q1).*sin(q3).*sin(q5).*sqrt(-sqrt(2.0)+2.0).*(3.0./4.0e+1)+(cos(q2).*cos(q4).*cos(q5).*sin(q1))./1.0e+1+(cos(q1).*cos(q3).*cos(q5).*sin(q4))./1.0e+1-(cos(q3).*sin(q1).*sin(q2).*sin(q5))./1.0e+1+cos(q2).*cos(q4).*cos(q5).*sin(q1).*sqrt(-sqrt(2.0)+2.0).*(3.0./4.0e+1)+cos(q1).*cos(q3).*cos(q5).*sin(q4).*sqrt(-sqrt(2.0)+2.0).*(3.0./4.0e+1)-cos(q3).*sin(q1).*sin(q2).*sin(q5).*sqrt(-sqrt(2.0)+2.0).*(3.0./4.0e+1)+(cos(q5).*sin(q1).*sin(q2).*sin(q3).*sin(q4))./1.0e+1+cos(q1).*cos(q5).*cos(q6).*sin(q3).*sqrt(sqrt(2.0)+2.0).*(3.0./4.0e+1);
    et42 = cos(q5).*sin(q1).*sin(q2).*sin(q3).*sin(q4).*sqrt(-sqrt(2.0)+2.0).*(3.0./4.0e+1)-cos(q3).*cos(q5).*cos(q6).*sin(q1).*sin(q2).*sqrt(sqrt(2.0)+2.0).*(3.0./4.0e+1)-cos(q2).*cos(q4).*cos(q6).*sin(q1).*sin(q5).*sqrt(sqrt(2.0)+2.0).*(3.0./4.0e+1)-cos(q1).*cos(q3).*cos(q6).*sin(q4).*sin(q5).*sqrt(sqrt(2.0)+2.0).*(3.0./4.0e+1)-cos(q6).*sin(q1).*sin(q2).*sin(q3).*sin(q4).*sin(q5).*sqrt(sqrt(2.0)+2.0).*(3.0./4.0e+1);
    et43 = sin(q1).*sin(q3).*sin(q5).*sin(q6).*sqrt(sqrt(2.0)+2.0).*(-3.0./4.0e+1)+cos(q1).*cos(q2).*cos(q6).*sin(q4).*sqrt(sqrt(2.0)+2.0).*(3.0./4.0e+1)+cos(q3).*cos(q4).*cos(q6).*sin(q1).*sqrt(sqrt(2.0)+2.0).*(3.0./4.0e+1)+cos(q1).*cos(q2).*cos(q4).*cos(q5).*sin(q6).*sqrt(sqrt(2.0)+2.0).*(3.0./4.0e+1)-cos(q1).*cos(q4).*cos(q6).*sin(q2).*sin(q3).*sqrt(sqrt(2.0)+2.0).*(3.0./4.0e+1)-cos(q1).*cos(q3).*sin(q2).*sin(q5).*sin(q6).*sqrt(sqrt(2.0)+2.0).*(3.0./4.0e+1)-cos(q3).*cos(q5).*sin(q1).*sin(q4).*sin(q6).*sqrt(sqrt(2.0)+2.0).*(3.0./4.0e+1);
    et44 = cos(q1).*cos(q5).*sin(q2).*sin(q3).*sin(q4).*sin(q6).*sqrt(sqrt(2.0)+2.0).*(3.0./4.0e+1);
    et45 = cos(q1).*cos(q3).*cos(q4).*cos(q6).*sqrt(sqrt(2.0)+2.0).*(3.0./4.0e+1)-cos(q2).*cos(q6).*sin(q1).*sin(q4).*sqrt(sqrt(2.0)+2.0).*(3.0./4.0e+1)-cos(q1).*sin(q3).*sin(q5).*sin(q6).*sqrt(sqrt(2.0)+2.0).*(3.0./4.0e+1)-cos(q2).*cos(q4).*cos(q5).*sin(q1).*sin(q6).*sqrt(sqrt(2.0)+2.0).*(3.0./4.0e+1)-cos(q1).*cos(q3).*cos(q5).*sin(q4).*sin(q6).*sqrt(sqrt(2.0)+2.0).*(3.0./4.0e+1)+cos(q4).*cos(q6).*sin(q1).*sin(q2).*sin(q3).*sqrt(sqrt(2.0)+2.0).*(3.0./4.0e+1)+cos(q3).*sin(q1).*sin(q2).*sin(q5).*sin(q6).*sqrt(sqrt(2.0)+2.0).*(3.0./4.0e+1);
    et46 = cos(q5).*sin(q1).*sin(q2).*sin(q3).*sin(q4).*sin(q6).*sqrt(sqrt(2.0)+2.0).*(-3.0./4.0e+1);
    mt5 = [et20+et21+et22,et17+et18+et19,0.0,0.0,0.0,1.0,(sin(q1).*(et27+et28))./4.0e+1,cos(q1).*(et25+et26).*(-1.0./4.0e+1),et23+et24,cos(q1),sin(q1),0.0,et31+et32,et29+et30,(cos(q2).*(cos(q3).*cos(q4).*2.0e+1-cos(q3).*sin(q4).*4.0-cos(q5).*sin(q3).*4.0-cos(q5).*sin(q3).*sqrt(-sqrt(2.0)+2.0).*3.0+cos(q3).*sin(q4).*sin(q5).*4.0+cos(q3).*cos(q4).*sin(q6).*sqrt(sqrt(2.0)+2.0).*3.0+cos(q6).*sin(q3).*sin(q5).*sqrt(sqrt(2.0)+2.0).*3.0+cos(q3).*sin(q4).*sin(q5).*sqrt(-sqrt(2.0)+2.0).*3.0+cos(q3).*cos(q5).*cos(q6).*sin(q4).*sqrt(sqrt(2.0)+2.0).*3.0))./4.0e+1,cos(q2).*sin(q1),-cos(q1).*cos(q2)];
    mt6 = [-sin(q2),et37+et38,et35+et36,et33+et34,-cos(q1).*sin(q3)+cos(q3).*sin(q1).*sin(q2),-sin(q1).*sin(q3)-cos(q1).*cos(q3).*sin(q2),cos(q2).*cos(q3),et41+et42,et39+et40];
    mt7 = [cos(q2).*cos(q3).*sin(q5).*(-1.0./1.0e+1)-(cos(q4).*cos(q5).*sin(q2))./1.0e+1-cos(q2).*cos(q3).*sin(q5).*sqrt(-sqrt(2.0)+2.0).*(3.0./4.0e+1)-cos(q4).*cos(q5).*sin(q2).*sqrt(-sqrt(2.0)+2.0).*(3.0./4.0e+1)+(cos(q2).*cos(q5).*sin(q3).*sin(q4))./1.0e+1+cos(q2).*cos(q5).*sin(q3).*sin(q4).*sqrt(-sqrt(2.0)+2.0).*(3.0./4.0e+1)-cos(q2).*cos(q3).*cos(q5).*cos(q6).*sqrt(sqrt(2.0)+2.0).*(3.0./4.0e+1)+cos(q4).*cos(q6).*sin(q2).*sin(q5).*sqrt(sqrt(2.0)+2.0).*(3.0./4.0e+1)-cos(q2).*cos(q6).*sin(q3).*sin(q4).*sin(q5).*sqrt(sqrt(2.0)+2.0).*(3.0./4.0e+1)];
    mt8 = [cos(q1).*cos(q3).*cos(q4)-cos(q2).*sin(q1).*sin(q4)+cos(q4).*sin(q1).*sin(q2).*sin(q3),cos(q1).*cos(q2).*sin(q4)+cos(q3).*cos(q4).*sin(q1)-cos(q1).*cos(q4).*sin(q2).*sin(q3),sin(q2).*sin(q4)+cos(q2).*cos(q4).*sin(q3),et45+et46,et43+et44,cos(q6).*sin(q2).*sin(q4).*sqrt(sqrt(2.0)+2.0).*(3.0./4.0e+1)+cos(q2).*cos(q4).*cos(q6).*sin(q3).*sqrt(sqrt(2.0)+2.0).*(3.0./4.0e+1)+cos(q2).*cos(q3).*sin(q5).*sin(q6).*sqrt(sqrt(2.0)+2.0).*(3.0./4.0e+1)+cos(q4).*cos(q5).*sin(q2).*sin(q6).*sqrt(sqrt(2.0)+2.0).*(3.0./4.0e+1)-cos(q2).*cos(q5).*sin(q3).*sin(q4).*sin(q6).*sqrt(sqrt(2.0)+2.0).*(3.0./4.0e+1)];
    mt9 = [-cos(q1).*cos(q5).*sin(q3)+cos(q3).*cos(q5).*sin(q1).*sin(q2)+cos(q2).*cos(q4).*sin(q1).*sin(q5)+cos(q1).*cos(q3).*sin(q4).*sin(q5)+sin(q1).*sin(q2).*sin(q3).*sin(q4).*sin(q5),-cos(q5).*sin(q1).*sin(q3)-cos(q1).*cos(q3).*cos(q5).*sin(q2)-cos(q1).*cos(q2).*cos(q4).*sin(q5)+cos(q3).*sin(q1).*sin(q4).*sin(q5)-cos(q1).*sin(q2).*sin(q3).*sin(q4).*sin(q5),cos(q2).*cos(q3).*cos(q5)-cos(q4).*sin(q2).*sin(q5)+cos(q2).*sin(q3).*sin(q4).*sin(q5)];
    J = reshape([mt5,mt6,mt7,mt8,mt9],6,6);
end
end
